simulink model "ThreePhase_Inverter"  (R2023a)
settings: Solver=ode23t  StartTime=0.0  StopTime=0.1  MaxStep=1e-4  RelTol=1e-3
libraries: spsMosfetLib x12, spsSeriesRLCBranchLib x6, spsThreePhaseVIMeasurementLib x4, spsDCVoltageSourceLib x2, spsGroundLib x2, sps_lib x1
settings Model: Creator=Alielden  LastModifiedBy=Alielden

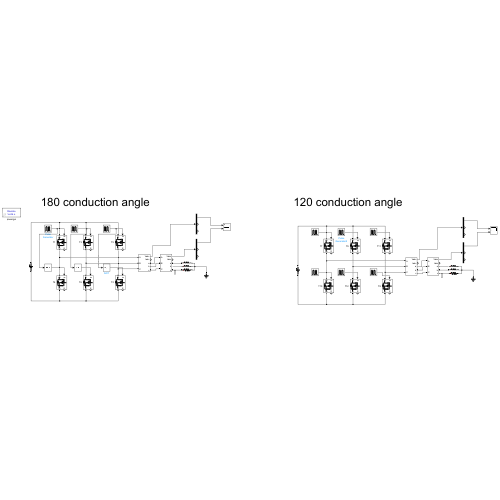
[thumbnail: Simulink's stored preview of the top-level diagram]
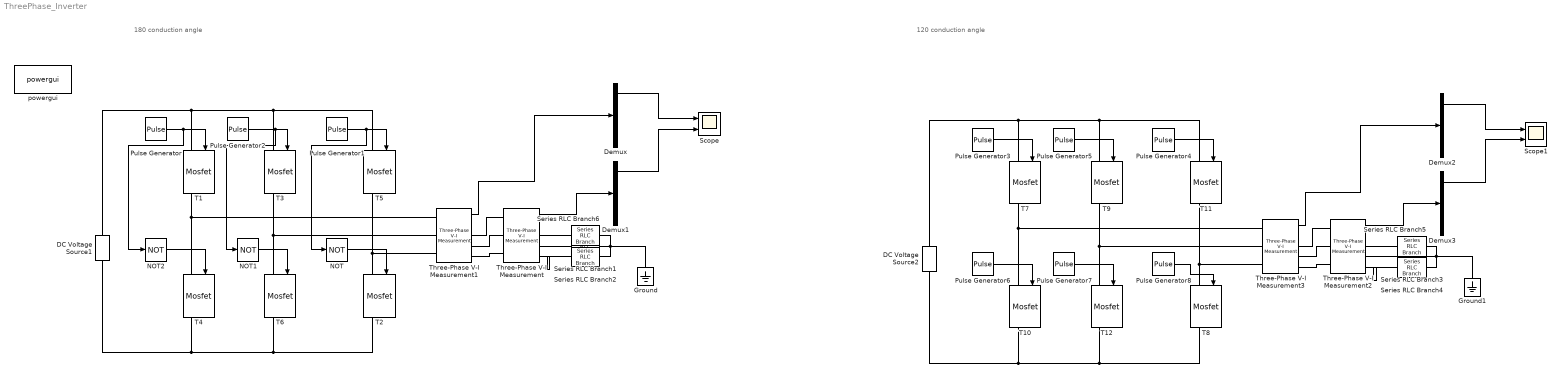
== system ThreePhase_Inverter ==
  note: 120 conduction angle
  note: 180 conduction angle
  DC Voltage Source1 : spsDCVoltageSourceLib/DC Voltage Source  Amplitude=100  Measurements=None
  DC Voltage Source2 : spsDCVoltageSourceLib/DC Voltage Source  Amplitude=100  Measurements=None
  Demux{,1..3} (4 alike) : Demux  Outputs=3
  Ground : spsGroundLib/Ground  LConnTagsString=a
  Ground1 : spsGroundLib/Ground  LConnTagsString=a
  NOT : Logic  Operator=NOT  AllPortsSameDT=off  OutDataTypeStr=boolean
  NOT1 : Logic  Operator=NOT  AllPortsSameDT=off  OutDataTypeStr=boolean
  NOT2 : Logic  Operator=NOT  AllPortsSameDT=off  OutDataTypeStr=boolean
  Pulse Generator : DiscretePulseGenerator  PulseType=Time based  Period=0.02  PulseWidth=50
  Pulse Generator1 : DiscretePulseGenerator  PulseType=Time based  Period=0.02  PulseWidth=50  PhaseDelay=(5-1)*60*0.02 / 360
  Pulse Generator2 : DiscretePulseGenerator  PulseType=Time based  Period=0.02  PulseWidth=50  PhaseDelay=(3-1)*60*0.02 / 360
  Pulse Generator3 : DiscretePulseGenerator  PulseType=Time based  Period=0.02  PulseWidth=100/3
  Pulse Generator4 : DiscretePulseGenerator  PulseType=Time based  Period=0.02  PulseWidth=100/3  PhaseDelay=(5-1)*60*0.02 / 360
  Pulse Generator5 : DiscretePulseGenerator  PulseType=Time based  Period=0.02  PulseWidth=100/3  PhaseDelay=(3-1)*60*0.02 / 360
  Pulse Generator6 : DiscretePulseGenerator  PulseType=Time based  Period=0.02  PulseWidth=100/3  PhaseDelay=(4-1)*60*0.02 / 360
  Pulse Generator7 : DiscretePulseGenerator  PulseType=Time based  Period=0.02  PulseWidth=100/3  PhaseDelay=(6-1)*60*0.02 / 360
  Pulse Generator8 : DiscretePulseGenerator  PulseType=Time based  Period=0.02  PulseWidth=100/3  PhaseDelay=(2-1)*60*0.02 / 360
  Scope : Scope  NumInputPorts=2
  Scope1 : Scope  NumInputPorts=2
  Series RLC Branch{1..6} (6 alike) : spsSeriesRLCBranchLib/Series RLC Branch  LConnTagsString=__new0  RConnTagsString=__new0  BranchType=R  Resistance=10  Inductance=1e-3  SetiL0=off  InitialCurrent=0  Capacitance=1e-6  Setx0=off  InitialVoltage=0  Measurements=None
  T{1..12} (12 alike) : spsMosfetLib/Mosfet  Ron=0.1  Lon=0  Rd=0.01  Vfd=0  IC=0  Rs=1e5  Cs=inf  Measurements=on
  Three-Phase V-I Measurement : spsThreePhaseVIMeasurementLib/Three-Phase V-I Measurement  VoltageMeasurement=phase-to-phase  SetLabelV=off  LabelV=Vab  Vpu=off  VpuLL=off  CurrentMeasurement=yes  SetLabelI=off  LabelI=Iabc  Ipu=off  Pbase=100e6  Vbase=500e3  OutputType=Complex  PhasorSimulation=off  PSBequivalent=0
  Three-Phase V-I Measurement1 : spsThreePhaseVIMeasurementLib/Three-Phase V-I Measurement  VoltageMeasurement=phase-to-ground  SetLabelV=off  LabelV=Van  Vpu=off  VpuLL=off  CurrentMeasurement=yes  SetLabelI=off  LabelI=Iabc  Ipu=off  Pbase=100e6  Vbase=500e3  OutputType=Complex  PhasorSimulation=off  PSBequivalent=0
  Three-Phase V-I Measurement2 : spsThreePhaseVIMeasurementLib/Three-Phase V-I Measurement  VoltageMeasurement=phase-to-phase  SetLabelV=off  LabelV=Vab  Vpu=off  VpuLL=off  CurrentMeasurement=yes  SetLabelI=off  LabelI=Iabc  Ipu=off  Pbase=100e6  Vbase=500e3  OutputType=Complex  PhasorSimulation=off  PSBequivalent=0
  Three-Phase V-I Measurement3 : spsThreePhaseVIMeasurementLib/Three-Phase V-I Measurement  VoltageMeasurement=phase-to-ground  SetLabelV=off  LabelV=Van  Vpu=off  VpuLL=off  CurrentMeasurement=yes  SetLabelI=off  LabelI=Iabc  Ipu=off  Pbase=100e6  Vbase=500e3  OutputType=Complex  PhasorSimulation=off  PSBequivalent=0
  powergui : sps_lib/powergui  Priority=1  SimulationMode=Discrete  SampleTime=1e-6  frequency=60  Iterations=50  frequencyindice=0  Pbase=100e6  ErrMax=1e-4  UnitsV=kV  UnitsW=MW  buscounter=0  FunctionMessages=off  echomessages=off  EnableUseOfTLC=off  CurrentSourceSwitches=off  DisableSnubberDevices=off  DisableRonSwitches=off  DisableVfSwitches=off  DisplayEquations=off  AutomaticDiscreteSolvers=off  SolverType=Tustin/Backward Euler (TBE)  Interpol=off  ExternalGateDelay=off  methode=off  Ts=100  x0status=blocks  SPID=on  SwTol=0  HookPort=off  NonlinearTolerance=1e-4  nMaxIteration=100  ContinueOnMaxIteration=off  RestoreLinks=warning  ResistiveCurrentMeasurement=off  Frange=[0:2:500]  Ylog=off  Xlog=on  ShowGrid=off  save=off  variable=ZData  structure=0  ZoomFFT=off  StartTime=0.0  cycles=1  DisplayStyle=1  fundamental=60  FreqAxis=off  MaxFrequency=1000  frequencyindicesteady=1  RmsSteady=1  display=off
  wires:
  Three-Phase V-I Measurement1/1 -> Demux/1
  Demux/1 -> Scope/1
  Three-Phase V-I Measurement/1 -> Demux1/1
  Demux1/1 -> Scope/2
  Pulse Generator/1 -> NOT2/1, T1/1
  NOT/1 -> T2/1
  Pulse Generator2/1 -> NOT1/1, T3/1
  Pulse Generator1/1 -> NOT/1, T5/1
  NOT2/1 -> T4/1
  NOT1/1 -> T6/1
  Pulse Generator7/1 -> T12/1
  Pulse Generator6/1 -> T10/1
  Pulse Generator8/1 -> T8/1
  Three-Phase V-I Measurement2/1 -> Demux3/1
  Pulse Generator5/1 -> T9/1
  Pulse Generator4/1 -> T11/1
  Three-Phase V-I Measurement3/1 -> Demux2/1
  Pulse Generator3/1 -> T7/1
  Demux2/1 -> Scope1/1
  Demux3/1 -> Scope1/2
  connections:
  T6/LConn1 -- Three-Phase V-I Measurement1/LConn2 -- T3/RConn1
  DC Voltage Source1/RConn1 -- T1/LConn1 -- T5/LConn1 -- T3/LConn1
  T6/RConn1 -- T2/RConn1 -- T4/RConn1 -- DC Voltage Source1/LConn1
  T4/LConn1 -- Three-Phase V-I Measurement1/LConn1 -- T1/RConn1
  T2/LConn1 -- Three-Phase V-I Measurement1/LConn3 -- T5/RConn1
  Series RLC Branch6/RConn1 -- Ground/LConn1 -- Series RLC Branch1/RConn1 -- Series RLC Branch2/RConn1
  Three-Phase V-I Measurement/RConn1 -- Series RLC Branch6/LConn1
  Three-Phase V-I Measurement/RConn2 -- Series RLC Branch1/LConn1
  Three-Phase V-I Measurement/RConn3 -- Series RLC Branch2/LConn1
  Three-Phase V-I Measurement1/RConn1 -- Three-Phase V-I Measurement/LConn1
  Three-Phase V-I Measurement1/RConn2 -- Three-Phase V-I Measurement/LConn2
  Three-Phase V-I Measurement1/RConn3 -- Three-Phase V-I Measurement/LConn3
  Series RLC Branch5/RConn1 -- Ground1/LConn1 -- Series RLC Branch3/RConn1 -- Series RLC Branch4/RConn1
  T10/LConn1 -- Three-Phase V-I Measurement3/LConn1 -- T7/RConn1
  T12/LConn1 -- Three-Phase V-I Measurement3/LConn2 -- T9/RConn1
  DC Voltage Source2/LConn1 -- T10/RConn1 -- T8/RConn1 -- T12/RConn1
  T11/RConn1 -- T8/LConn1 -- Three-Phase V-I Measurement3/LConn3
  DC Voltage Source2/RConn1 -- T7/LConn1 -- T11/LConn1 -- T9/LConn1
  Three-Phase V-I Measurement3/RConn2 -- Three-Phase V-I Measurement2/LConn2
  Three-Phase V-I Measurement2/RConn2 -- Series RLC Branch3/LConn1
  Three-Phase V-I Measurement3/RConn3 -- Three-Phase V-I Measurement2/LConn3
  Three-Phase V-I Measurement2/RConn3 -- Series RLC Branch4/LConn1
  Three-Phase V-I Measurement3/RConn1 -- Three-Phase V-I Measurement2/LConn1
  Three-Phase V-I Measurement2/RConn1 -- Series RLC Branch5/LConn1
